simulink model "cruise_control"  (R2017b)
settings: Solver=VariableStepAuto  StartTime=0.0  StopTime=10.0  RelTol=1e-3
values from neighbouring files (symbols this model uses):
  Ki = 1    [cruise_control.mat]    (also in cruise_control_external.mat = 0.002; cruise_control_sim.mat = 0.002)
  Kp = 1    [cruise_control.mat]    (also in cruise_control_external.mat = 0.4; cruise_control_sim.mat = 0.4)
settings Model: Creator=Rehaan M. Bhimani  LastModifiedBy=Rehaan M. Bhimani

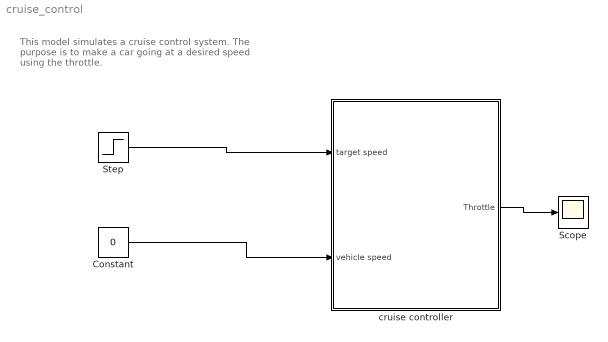
== system cruise_control ==
  note: This model simulates a cruise control system.
      | The purpose is to make a car going at a desired
      | speed using the throttle.
  Constant : Constant  Value=0
  Scope : Scope
  Step : Step  After=0.1  SampleTime=0
  "cruise controller " : Subsystem
  wires:
  Step/1 -> "cruise controller "/1(target speed)
  Constant/1 -> "cruise controller "/2(vehicle speed)
  "cruise controller "/1("Throttle ") -> Scope/1

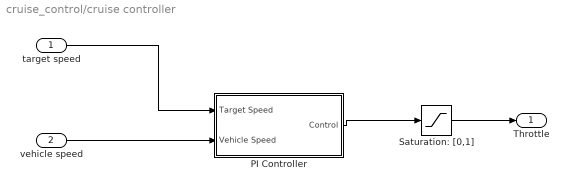
== system cruise_control/cruise controller  ==
  target speed : Inport
  vehicle speed : Inport  Port=2
  PI Controller : Subsystem
  Saturation: [0,1] : Saturate  UpperLimit=1  LowerLimit=0
  "Throttle " : Outport
  wires:
  Saturation: [0,1]/1 -> "Throttle "/1
  target speed/1 -> PI Controller/1(Target Speed)
  vehicle speed/1 -> PI Controller/2(Vehicle Speed)
  PI Controller/1(Control) -> Saturation: [0,1]/1

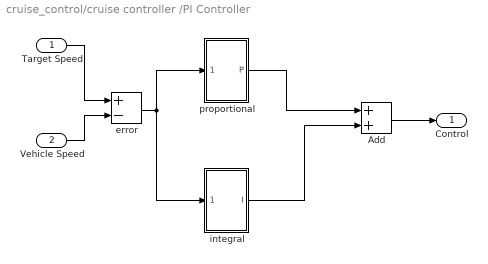
== system cruise_control/cruise controller /PI Controller ==
  Target Speed : Inport
  Vehicle Speed : Inport  Port=2
  Add : Sum
  error : Sum  Inputs=+-
  integral : Subsystem
  proportional : Subsystem
  Control : Outport
  wires:
  Add/1 -> Control/1
  Vehicle Speed/1 -> error/2
  integral/1(I) -> Add/2
  Target Speed/1 -> error/1
  error/1 -> integral/1(error), proportional/1(error)
  proportional/1("P ") -> Add/1

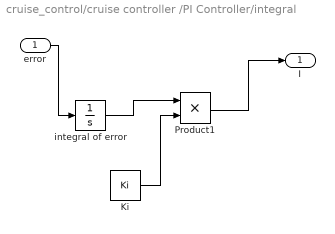
== system cruise_control/cruise controller /PI Controller/integral ==
  error : Inport
  Ki : Constant  Value=Ki
  Product1 : Product
  integral of error : Integrator
  I : Outport
  wires:
  integral of error/1 -> Product1/1
  Ki/1 -> Product1/2
  error/1 -> integral of error/1
  Product1/1 -> I/1

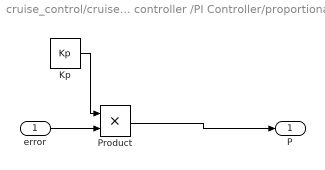
== system cruise_control/cruise controller /PI Controller/proportional ==
  error : Inport
  "Kp " : Constant  Value=Kp
  Product : Product
  "P " : Outport
  wires:
  Product/1 -> "P "/1
  error/1 -> Product/2
  "Kp "/1 -> Product/1
